simulink model "Factorial"  (R2016b)
settings: Solver=FixedStepDiscrete  StartTime=0.0  StopTime=10.0  RelTol=1e-3
settings Model: Creator=3essawy  LastModifiedBy=3essawy
settings OptimizationCC: DefaultParameterBehavior=Inlined
settings DebuggingCC: ParameterTunabilityLossMsg=error
settings RTWCC: SystemTargetFile=ert.tlc  GenCodeOnly=on  TemplateMakefile=ert_default_tmf  Description=Embedded Coder  GenerateReport=on  IncludeHyperlinkInReport=on  LaunchReport=on  GenerateTraceInfo=on  GenerateTraceReport=on  GenerateTraceReportSl=on  GenerateTraceReportSf=on  GenerateTraceReportEml=on
settings CodeAppCC: ForceParamTrailComments=on  IgnoreCustomStorageClasses=off  OperatorAnnotations=on  SimulinkDataObjDesc=on  SFDataObjDesc=on  MATLABFcnDesc=on  InsertBlockDesc=on  MATLABSourceComments=on
settings ERTTargetCC: TargetLangStandard=C99 (ISO)  GenerateSampleERTMain=on  InlinedParameterPlacement=NonHierarchical  ERTCustomFileTemplate=example_file_process.tlc  EnableUserReplacementTypes=on

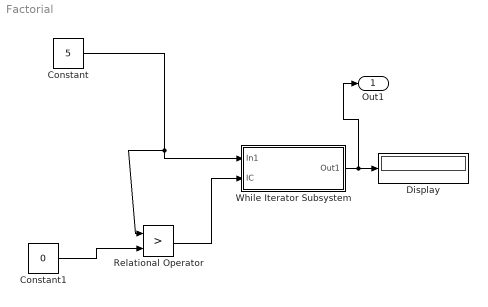
== system Factorial ==
  Constant : Constant  Value=5
  Constant1 : Constant  Value=0
  Display : Display
  Relational Operator : RelationalOperator  Operator=>  OutDataTypeStr=boolean  RndMeth=Simplest
  While Iterator Subsystem : Subsystem  TreatAsAtomicUnit=on
  Out1 : Outport
  wires:
  While Iterator Subsystem/1(Out1) -> Out1/1, Display/1
  Relational Operator/1 -> While Iterator Subsystem/2(IC)
  Constant1/1 -> Relational Operator/2
  Constant/1 -> Relational Operator/1, While Iterator Subsystem/1(In1)

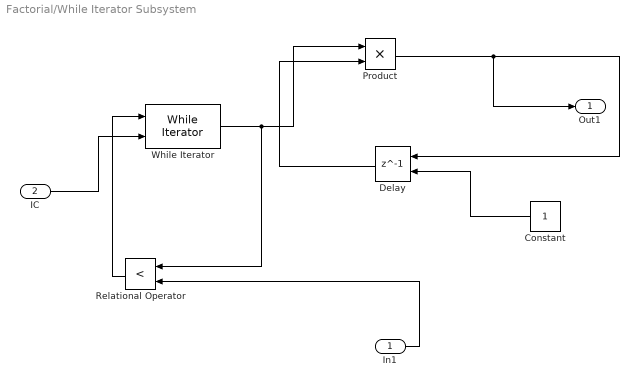
== system Factorial/While Iterator Subsystem ==
  In1 : Inport
  IC : Inport  Port=2
  Constant : Constant
  Delay : Delay  DelayLength=1  InitialConditionSource=Input port  InitialCondition=1
      settings: InputPortMap=u0,p4
  Product : Product
  Relational Operator : RelationalOperator  Operator=<  OutDataTypeStr=boolean  RndMeth=Simplest
  While Iterator : WhileIterator  MaxIters=20  ResetStates=reset  ShowIterationPort=on
  Out1 : Outport
  wires:
  IC/1 -> While Iterator/2
  Relational Operator/1 -> While Iterator/1
  While Iterator/1 -> Relational Operator/1, Product/1
  Product/1 -> Out1/1, Delay/1
  Delay/1 -> Product/2
  Constant/1 -> Delay/2
  In1/1 -> Relational Operator/2
